simulink model "MultipleAgentsChoice_NoVR"  (Simulink 7.5)
settings: Solver=ode45  StartTime=0.0  StopTime=1000  RelTol=1e-4  AbsTol=1e-4
libraries: simulink x64
(part 5 of 6)

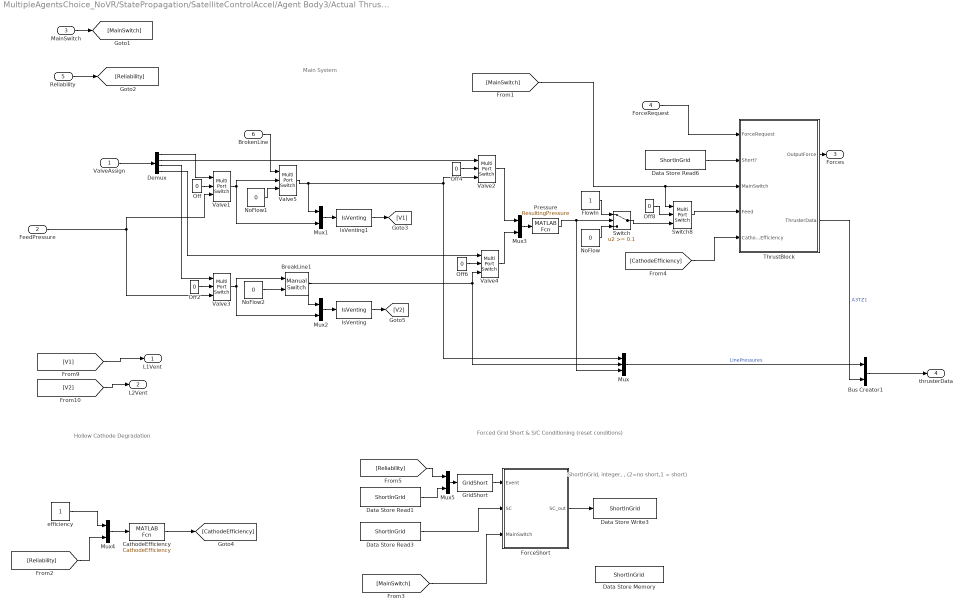
== system MultipleAgentsChoice_NoVR/StatePropagation/SatelliteControlAccel/Agent Body3/Actual Thruster response/Zthruster1/Thruster1 ==
  note: Forced Grid Short & S/C Conditioning (reset conditions)
  note: ShortInGrid, integer, , (2=no short,1 = short)
  note: Hollow Cathode Degradation
  note: Main System
  ValveAssign : Inport  OutDataType=sfix(16)  OutScaling=2^0
  FeedPressure : Inport  Port=2  OutDataType=sfix(16)  OutScaling=2^0
  MainSwitch : Inport  Port=3  OutDataType=sfix(16)  OutScaling=2^0
  ForceRequest : Inport  Port=4  OutDataType=sfix(16)  OutScaling=2^0
  Reliability : Inport  Port=5  OutDataType=sfix(16)  OutScaling=2^0
  BrokenLine : Inport  Port=6  OutDataType=sfix(16)  OutScaling=2^0
  BreakLine1 : simulink/Signal Routing/Manual Switch  SystemSampleTime=-1  sw=1  action=0  varsize=off
  Bus Creator1 : BusCreator  Inputs=2
  CathodeEfficiency : MATLABFcn  MATLABFcn=CathodeEfficiency  OutputDimensions=1
  Data Store Memory : DataStoreMemory  DataStoreName=ShortInGrid  ReadBeforeWriteMsg=warning  WriteAfterWriteMsg=warning  WriteAfterReadMsg=warning  InitialValue=2  OutDataType=sfix(16)  OutScaling=2^0
  Data Store Read1 : DataStoreRead  DataStoreName=ShortInGrid  SampleTime=0
  Data Store Read3 : DataStoreRead  DataStoreName=ShortInGrid  SampleTime=0
  Data Store Read6 : DataStoreRead  DataStoreName=ShortInGrid  SampleTime=0
  Data Store Write3 : DataStoreWrite  DataStoreName=ShortInGrid  SampleTime=-1
  Demux : Demux
  FlowIn : Constant  OutDataType=sfix(16)  OutScaling=2^0
  ForceShort : Subsystem
  GridShort : MATLABFcn  MATLABFcn=GridShort  OutputDimensions=1
  IsVenting : MATLABFcn  MATLABFcn=IsVenting  OutputDimensions=1
  IsVenting1 : MATLABFcn  MATLABFcn=IsVenting  OutputDimensions=1
  Mux : Mux  Inputs=3
  Mux{1..5} (5 alike) : Mux  Inputs=2
  NoFlow : Constant  Value=0  OutDataType=sfix(16)  OutScaling=2^0
  NoFlow1 : Constant  Value=0  OutDataType=sfix(16)  OutScaling=2^0
  NoFlow2 : Constant  Value=0  OutDataType=sfix(16)  OutScaling=2^0
  Off{,2,4,6,8} (5 alike) : Constant  Value=0  OutDataType=sfix(16)  OutScaling=2^0
  Pressure : MATLABFcn  MATLABFcn=ResultingPressure
  Switch : Switch  Threshold=0.1
  Switch8 : MultiPortSwitch  Inputs=2  zeroidx=off
  ThrustBlock : Subsystem
  Valve{1..5} (5 alike) : MultiPortSwitch  Inputs=2  zeroidx=off
  efficiency : Constant  OutDataType=sfix(16)  OutScaling=2^0
  L1Vent : Outport  OutDataType=sfix(16)  OutScaling=2^0
  L2Vent : Outport  Port=2  OutDataType=sfix(16)  OutScaling=2^0
  Forces : Outport  Port=3  OutDataType=sfix(16)  OutScaling=2^0
  thrusterData : Outport  Port=4  OutDataType=sfix(16)  OutScaling=2^0
  wires:
  ForceShort/1(SC_out) -> Data Store Write3/1
  GridShort/1 -> ForceShort/1(Event)
  Data Store Read3/1 -> ForceShort/2(SC)
  [MainSwitch] -> ForceShort/3(MainSwitch)
  Valve1/1 -> Mux1/2, Valve5/2
  Valve2/1 -> Mux3/1
  Mux3/1 -> Pressure/1
  Valve5/1 -> Mux1/1, Valve2/3, Mux/1
  FlowIn/1 -> Switch/1
  NoFlow/1 -> Switch/3
  Switch8/1 -> ThrustBlock/4(Feed)
  Data Store Read6/1 -> ThrustBlock/2(Short?)
  ValveAssign/1 -> Demux/1
  Demux/1 -> Valve1/1
  Demux/2 -> Valve2/1
  Demux/3 -> Valve3/1
  Demux/4 -> Valve4/1
  ThrustBlock/2(ThrusterData) -> Bus Creator1/2  "A3TZ1"
  ThrustBlock/1(OutputForce) -> Forces/1
  NoFlow1/1 -> Valve5/3
  Off/1 -> Valve1/2
  Off4/1 -> Valve2/2
  Off2/1 -> Valve3/2
  Off6/1 -> Valve4/2
  Off8/1 -> Switch8/2
  Switch/1 -> Switch8/3
  Mux/1 -> Bus Creator1/1  "LinePressures"
  NoFlow2/1 -> BreakLine1/2
  Valve3/1 -> BreakLine1/1, Mux2/2
  BreakLine1/1 -> Mux2/1, Valve4/3, Mux/2
  [CathodeEfficiency] -> ThrustBlock/5(CathodeEfficiency)
  ForceRequest/1 -> ThrustBlock/1(ForceRequest)
  Bus Creator1/1 -> thrusterData/1
  Mux1/1 -> IsVenting1/1
  Mux2/1 -> IsVenting/1
  Pressure/1 -> Switch/2, Mux/3
  IsVenting1/1 -> [V1]
  IsVenting/1 -> [V2]
  FeedPressure/1 -> Valve1/3, Valve3/3
  MainSwitch/1 -> [MainSwitch]
  Valve4/1 -> Mux3/2
  [MainSwitch] -> ThrustBlock/3(MainSwitch), Switch8/1
  Reliability/1 -> [Reliability]
  efficiency/1 -> Mux4/1
  [Reliability] -> Mux4/2
  Mux4/1 -> CathodeEfficiency/1
  CathodeEfficiency/1 -> [CathodeEfficiency]
  Mux5/1 -> GridShort/1
  Data Store Read1/1 -> Mux5/2
  [Reliability] -> Mux5/1
  BrokenLine/1 -> Valve5/1
  [V1] -> L1Vent/1
  [V2] -> L2Vent/1

== system MultipleAgentsChoice_NoVR/StatePropagation/SatelliteControlAccel/Agent Body1/Actual Thruster response/XYZthruster/Thruster1/ForceShort ==
  note: Detect event and introduce short, otherwise pass through current result of short status
  Event : Inport  OutDataType=sfix(16)  OutScaling=2^0
  SC : Inport  Port=2  OutDataType=sfix(16)  OutScaling=2^0
  MainSwitch : Inport  Port=3  OutDataType=sfix(16)  OutScaling=2^0
  Constant : Constant  OutDataType=sfix(16)  OutScaling=2^0
  Data Type Conversion : DataTypeConversion  OutDataType=sfix(16)  OutScaling=2^0
  Detect Increase : simulink/Logic and Bit Operations/Detect Increase  SystemSampleTime=-1  vinit=0
  Multiport Switch : MultiPortSwitch  DataPortOrder=Zero-based contiguous  Inputs=2  zeroidx=on
  S/C Conditioning : Subsystem
  SC_out : Outport  OutDataType=sfix(16)  OutScaling=2^0
  wires:
  Event/1 -> Detect Increase/1
  Detect Increase/1 -> Data Type Conversion/1
  S/C Conditioning/1(Short?) -> SC_out/1
  MainSwitch/1 -> S/C Conditioning/2(MainSwitch)
  Data Type Conversion/1 -> Multiport Switch/1
  SC/1 -> Multiport Switch/2
  Constant/1 -> Multiport Switch/3
  Multiport Switch/1 -> S/C Conditioning/1(SC)

== system MultipleAgentsChoice_NoVR/StatePropagation/SatelliteControlAccel/Agent Body1/Actual Thruster response/XYZthruster/Thruster1/ThrustBlock ==
  ForceRequest : Inport  OutDataType=sfix(16)  OutScaling=2^0
  Short? : Inport  Port=2  OutDataType=sfix(16)  OutScaling=2^0
  MainSwitch : Inport  Port=3  OutDataType=sfix(16)  OutScaling=2^0
  Feed : Inport  Port=4  OutDataType=sfix(16)  OutScaling=2^0
  CathodeEfficiency : Inport  Port=5  OutDataType=sfix(16)  OutScaling=2^0
  ActiveThruster (logical) : Subsystem
  Bus Creator : BusCreator  Inputs=2
  Product : Product  OutDataType=sfix(16)  OutScaling=2^0  RndMeth=Zero
  Product1 : Product  OutDataType=sfix(16)  OutScaling=2^0  RndMeth=Zero
  Voltage/Current : Subsystem
  OutputForce : Outport  OutDataType=sfix(16)  OutScaling=2^0
  ThrusterData : Outport  Port=2  OutDataType=sfix(16)  OutScaling=2^0
  wires:
  MainSwitch/1 -> ActiveThruster (logical)/2(ThrusterOn?), Voltage/Current/2(MainSwitch)
  Short?/1 -> ActiveThruster (logical)/1(Short?), Voltage/Current/1(Short?)
  Feed/1 -> Voltage/Current/3(Feed?), ActiveThruster (logical)/3(Feed?)
  Voltage/Current/1(Voltage) -> Bus Creator/1  "voltage"
  Voltage/Current/2(Current) -> Bus Creator/2  "current"
  Bus Creator/1 -> ThrusterData/1
  ActiveThruster (logical)/1(Active) -> Product/1
  ForceRequest/1 -> [ForceRequest]
  CathodeEfficiency/1 -> [CathodeEfficiency]
  Product1/1 -> OutputForce/1
  [ForceRequest] -> Product/2
  Product/1 -> Product1/1
  [CathodeEfficiency] -> Product1/2

== system MultipleAgentsChoice_NoVR/StatePropagation/SatelliteControlAccel/Agent Body1/Actual Thruster response/Xthruster/Thruster1/ForceShort ==
  note: Detect event and introduce short, otherwise pass through current result of short status
  Event : Inport  OutDataType=sfix(16)  OutScaling=2^0
  SC : Inport  Port=2  OutDataType=sfix(16)  OutScaling=2^0
  MainSwitch : Inport  Port=3  OutDataType=sfix(16)  OutScaling=2^0
  Constant : Constant  OutDataType=sfix(16)  OutScaling=2^0
  Data Type Conversion : DataTypeConversion  OutDataType=sfix(16)  OutScaling=2^0
  Detect Increase : simulink/Logic and Bit Operations/Detect Increase  SystemSampleTime=-1  vinit=0
  Multiport Switch : MultiPortSwitch  DataPortOrder=Zero-based contiguous  Inputs=2  zeroidx=on
  S/C Conditioning : Subsystem
  SC_out : Outport  OutDataType=sfix(16)  OutScaling=2^0
  wires:
  Multiport Switch/1 -> S/C Conditioning/1(SC)
  Constant/1 -> Multiport Switch/3
  SC/1 -> Multiport Switch/2
  Data Type Conversion/1 -> Multiport Switch/1
  MainSwitch/1 -> S/C Conditioning/2(MainSwitch)
  S/C Conditioning/1(Short?) -> SC_out/1
  Detect Increase/1 -> Data Type Conversion/1
  Event/1 -> Detect Increase/1

== system MultipleAgentsChoice_NoVR/StatePropagation/SatelliteControlAccel/Agent Body1/Actual Thruster response/Xthruster/Thruster1/ThrustBlock ==
  ForceRequest : Inport  OutDataType=sfix(16)  OutScaling=2^0
  Short? : Inport  Port=2  OutDataType=sfix(16)  OutScaling=2^0
  MainSwitch : Inport  Port=3  OutDataType=sfix(16)  OutScaling=2^0
  Feed : Inport  Port=4  OutDataType=sfix(16)  OutScaling=2^0
  CathodeEfficiency : Inport  Port=5  OutDataType=sfix(16)  OutScaling=2^0
  ActiveThruster (logical) : Subsystem
  Bus Creator : BusCreator  Inputs=2
  Product : Product  OutDataType=sfix(16)  OutScaling=2^0  RndMeth=Zero
  Product1 : Product  OutDataType=sfix(16)  OutScaling=2^0  RndMeth=Zero
  Voltage/Current : Subsystem
  OutputForce : Outport  OutDataType=sfix(16)  OutScaling=2^0
  ThrusterData : Outport  Port=2  OutDataType=sfix(16)  OutScaling=2^0
  wires:
  [CathodeEfficiency] -> Product1/2
  Product/1 -> Product1/1
  [ForceRequest] -> Product/2
  CathodeEfficiency/1 -> [CathodeEfficiency]
  ForceRequest/1 -> [ForceRequest]
  ActiveThruster (logical)/1(Active) -> Product/1
  Bus Creator/1 -> ThrusterData/1
  Voltage/Current/2(Current) -> Bus Creator/2  "current"
  Voltage/Current/1(Voltage) -> Bus Creator/1  "voltage"
  Feed/1 -> ActiveThruster (logical)/3(Feed?), Voltage/Current/3(Feed?)
  Short?/1 -> Voltage/Current/1(Short?), ActiveThruster (logical)/1(Short?)
  MainSwitch/1 -> Voltage/Current/2(MainSwitch), ActiveThruster (logical)/2(ThrusterOn?)
  Product1/1 -> OutputForce/1

== system MultipleAgentsChoice_NoVR/StatePropagation/SatelliteControlAccel/Agent Body1/Actual Thruster response/Ythruster1/Thruster1/ForceShort ==
  note: Detect event and introduce short, otherwise pass through current result of short status
  Event : Inport  OutDataType=sfix(16)  OutScaling=2^0
  SC : Inport  Port=2  OutDataType=sfix(16)  OutScaling=2^0
  MainSwitch : Inport  Port=3  OutDataType=sfix(16)  OutScaling=2^0
  Constant : Constant  OutDataType=sfix(16)  OutScaling=2^0
  Data Type Conversion : DataTypeConversion  OutDataType=sfix(16)  OutScaling=2^0
  Detect Increase : simulink/Logic and Bit Operations/Detect Increase  SystemSampleTime=-1  vinit=0
  Multiport Switch : MultiPortSwitch  DataPortOrder=Zero-based contiguous  Inputs=2  zeroidx=on
  S/C Conditioning : Subsystem
  SC_out : Outport  OutDataType=sfix(16)  OutScaling=2^0
  wires:
  Event/1 -> Detect Increase/1
  Detect Increase/1 -> Data Type Conversion/1
  S/C Conditioning/1(Short?) -> SC_out/1
  MainSwitch/1 -> S/C Conditioning/2(MainSwitch)
  Data Type Conversion/1 -> Multiport Switch/1
  SC/1 -> Multiport Switch/2
  Constant/1 -> Multiport Switch/3
  Multiport Switch/1 -> S/C Conditioning/1(SC)

== system MultipleAgentsChoice_NoVR/StatePropagation/SatelliteControlAccel/Agent Body1/Actual Thruster response/Ythruster1/Thruster1/ThrustBlock ==
  ForceRequest : Inport  OutDataType=sfix(16)  OutScaling=2^0
  Short? : Inport  Port=2  OutDataType=sfix(16)  OutScaling=2^0
  MainSwitch : Inport  Port=3  OutDataType=sfix(16)  OutScaling=2^0
  Feed : Inport  Port=4  OutDataType=sfix(16)  OutScaling=2^0
  CathodeEfficiency : Inport  Port=5  OutDataType=sfix(16)  OutScaling=2^0
  ActiveThruster (logical) : Subsystem
  Bus Creator : BusCreator  Inputs=2
  Product : Product  OutDataType=sfix(16)  OutScaling=2^0  RndMeth=Zero
  Product1 : Product  OutDataType=sfix(16)  OutScaling=2^0  RndMeth=Zero
  Voltage/Current : Subsystem
  OutputForce : Outport  OutDataType=sfix(16)  OutScaling=2^0
  ThrusterData : Outport  Port=2  OutDataType=sfix(16)  OutScaling=2^0
  wires:
  MainSwitch/1 -> ActiveThruster (logical)/2(ThrusterOn?), Voltage/Current/2(MainSwitch)
  Short?/1 -> ActiveThruster (logical)/1(Short?), Voltage/Current/1(Short?)
  Feed/1 -> Voltage/Current/3(Feed?), ActiveThruster (logical)/3(Feed?)
  Voltage/Current/1(Voltage) -> Bus Creator/1  "voltage"
  Voltage/Current/2(Current) -> Bus Creator/2  "current"
  Bus Creator/1 -> ThrusterData/1
  ActiveThruster (logical)/1(Active) -> Product/1
  ForceRequest/1 -> [ForceRequest]
  CathodeEfficiency/1 -> [CathodeEfficiency]
  Product1/1 -> OutputForce/1
  [ForceRequest] -> Product/2
  Product/1 -> Product1/1
  [CathodeEfficiency] -> Product1/2

== system MultipleAgentsChoice_NoVR/StatePropagation/SatelliteControlAccel/Agent Body1/Actual Thruster response/Zthruster1/Thruster1/ForceShort ==
  note: Detect event and introduce short, otherwise pass through current result of short status
  Event : Inport  OutDataType=sfix(16)  OutScaling=2^0
  SC : Inport  Port=2  OutDataType=sfix(16)  OutScaling=2^0
  MainSwitch : Inport  Port=3  OutDataType=sfix(16)  OutScaling=2^0
  Constant : Constant  OutDataType=sfix(16)  OutScaling=2^0
  Data Type Conversion : DataTypeConversion  OutDataType=sfix(16)  OutScaling=2^0
  Detect Increase : simulink/Logic and Bit Operations/Detect Increase  SystemSampleTime=-1  vinit=0
  Multiport Switch : MultiPortSwitch  DataPortOrder=Zero-based contiguous  Inputs=2  zeroidx=on
  S/C Conditioning : Subsystem
  SC_out : Outport  OutDataType=sfix(16)  OutScaling=2^0
  wires:
  Multiport Switch/1 -> S/C Conditioning/1(SC)
  Constant/1 -> Multiport Switch/3
  SC/1 -> Multiport Switch/2
  Data Type Conversion/1 -> Multiport Switch/1
  MainSwitch/1 -> S/C Conditioning/2(MainSwitch)
  S/C Conditioning/1(Short?) -> SC_out/1
  Detect Increase/1 -> Data Type Conversion/1
  Event/1 -> Detect Increase/1

== system MultipleAgentsChoice_NoVR/StatePropagation/SatelliteControlAccel/Agent Body1/Actual Thruster response/Zthruster1/Thruster1/ThrustBlock ==
  ForceRequest : Inport  OutDataType=sfix(16)  OutScaling=2^0
  Short? : Inport  Port=2  OutDataType=sfix(16)  OutScaling=2^0
  MainSwitch : Inport  Port=3  OutDataType=sfix(16)  OutScaling=2^0
  Feed : Inport  Port=4  OutDataType=sfix(16)  OutScaling=2^0
  CathodeEfficiency : Inport  Port=5  OutDataType=sfix(16)  OutScaling=2^0
  ActiveThruster (logical) : Subsystem
  Bus Creator : BusCreator  Inputs=2
  Product : Product  OutDataType=sfix(16)  OutScaling=2^0  RndMeth=Zero
  Product1 : Product  OutDataType=sfix(16)  OutScaling=2^0  RndMeth=Zero
  Voltage/Current : Subsystem
  OutputForce : Outport  OutDataType=sfix(16)  OutScaling=2^0
  ThrusterData : Outport  Port=2  OutDataType=sfix(16)  OutScaling=2^0
  wires:
  [CathodeEfficiency] -> Product1/2
  Product/1 -> Product1/1
  [ForceRequest] -> Product/2
  Product1/1 -> OutputForce/1
  CathodeEfficiency/1 -> [CathodeEfficiency]
  ForceRequest/1 -> [ForceRequest]
  ActiveThruster (logical)/1(Active) -> Product/1
  Bus Creator/1 -> ThrusterData/1
  Voltage/Current/2(Current) -> Bus Creator/2  "current"
  Voltage/Current/1(Voltage) -> Bus Creator/1  "voltage"
  Feed/1 -> ActiveThruster (logical)/3(Feed?), Voltage/Current/3(Feed?)
  Short?/1 -> Voltage/Current/1(Short?), ActiveThruster (logical)/1(Short?)
  MainSwitch/1 -> Voltage/Current/2(MainSwitch), ActiveThruster (logical)/2(ThrusterOn?)

== system MultipleAgentsChoice_NoVR/StatePropagation/SatelliteControlAccel/Agent Body2/Actual Thruster response/XYZthruster/Thruster1/ForceShort ==
  note: Detect event and introduce short, otherwise pass through current result of short status
  Event : Inport  OutDataType=sfix(16)  OutScaling=2^0
  SC : Inport  Port=2  OutDataType=sfix(16)  OutScaling=2^0
  MainSwitch : Inport  Port=3  OutDataType=sfix(16)  OutScaling=2^0
  Constant : Constant  OutDataType=sfix(16)  OutScaling=2^0
  Data Type Conversion : DataTypeConversion  OutDataType=sfix(16)  OutScaling=2^0
  Detect Increase : simulink/Logic and Bit Operations/Detect Increase  SystemSampleTime=-1  vinit=0
  Multiport Switch : MultiPortSwitch  DataPortOrder=Zero-based contiguous  Inputs=2  zeroidx=on
  S/C Conditioning : Subsystem
  SC_out : Outport  OutDataType=sfix(16)  OutScaling=2^0
  wires:
  Multiport Switch/1 -> S/C Conditioning/1(SC)
  Constant/1 -> Multiport Switch/3
  SC/1 -> Multiport Switch/2
  Data Type Conversion/1 -> Multiport Switch/1
  MainSwitch/1 -> S/C Conditioning/2(MainSwitch)
  S/C Conditioning/1(Short?) -> SC_out/1
  Detect Increase/1 -> Data Type Conversion/1
  Event/1 -> Detect Increase/1

== system MultipleAgentsChoice_NoVR/StatePropagation/SatelliteControlAccel/Agent Body2/Actual Thruster response/XYZthruster/Thruster1/ThrustBlock ==
  ForceRequest : Inport  OutDataType=sfix(16)  OutScaling=2^0
  Short? : Inport  Port=2  OutDataType=sfix(16)  OutScaling=2^0
  MainSwitch : Inport  Port=3  OutDataType=sfix(16)  OutScaling=2^0
  Feed : Inport  Port=4  OutDataType=sfix(16)  OutScaling=2^0
  CathodeEfficiency : Inport  Port=5  OutDataType=sfix(16)  OutScaling=2^0
  ActiveThruster (logical) : Subsystem
  Bus Creator : BusCreator  Inputs=2
  Product : Product  OutDataType=sfix(16)  OutScaling=2^0  RndMeth=Zero
  Product1 : Product  OutDataType=sfix(16)  OutScaling=2^0  RndMeth=Zero
  Voltage/Current : Subsystem
  OutputForce : Outport  OutDataType=sfix(16)  OutScaling=2^0
  ThrusterData : Outport  Port=2  OutDataType=sfix(16)  OutScaling=2^0
  wires:
  [CathodeEfficiency] -> Product1/2
  Product/1 -> Product1/1
  [ForceRequest] -> Product/2
  CathodeEfficiency/1 -> [CathodeEfficiency]
  ForceRequest/1 -> [ForceRequest]
  ActiveThruster (logical)/1(Active) -> Product/1
  Bus Creator/1 -> ThrusterData/1
  Voltage/Current/2(Current) -> Bus Creator/2  "current"
  Voltage/Current/1(Voltage) -> Bus Creator/1  "voltage"
  Feed/1 -> ActiveThruster (logical)/3(Feed?), Voltage/Current/3(Feed?)
  Short?/1 -> Voltage/Current/1(Short?), ActiveThruster (logical)/1(Short?)
  MainSwitch/1 -> Voltage/Current/2(MainSwitch), ActiveThruster (logical)/2(ThrusterOn?)
  Product1/1 -> OutputForce/1

== system MultipleAgentsChoice_NoVR/StatePropagation/SatelliteControlAccel/Agent Body2/Actual Thruster response/Xthruster/Thruster1/ForceShort ==
  note: Detect event and introduce short, otherwise pass through current result of short status
  Event : Inport  OutDataType=sfix(16)  OutScaling=2^0
  SC : Inport  Port=2  OutDataType=sfix(16)  OutScaling=2^0
  MainSwitch : Inport  Port=3  OutDataType=sfix(16)  OutScaling=2^0
  Constant : Constant  OutDataType=sfix(16)  OutScaling=2^0
  Data Type Conversion : DataTypeConversion  OutDataType=sfix(16)  OutScaling=2^0
  Detect Increase : simulink/Logic and Bit Operations/Detect Increase  SystemSampleTime=-1  vinit=0
  Multiport Switch : MultiPortSwitch  DataPortOrder=Zero-based contiguous  Inputs=2  zeroidx=on
  S/C Conditioning : Subsystem
  SC_out : Outport  OutDataType=sfix(16)  OutScaling=2^0
  wires:
  Event/1 -> Detect Increase/1
  Detect Increase/1 -> Data Type Conversion/1
  S/C Conditioning/1(Short?) -> SC_out/1
  MainSwitch/1 -> S/C Conditioning/2(MainSwitch)
  Data Type Conversion/1 -> Multiport Switch/1
  SC/1 -> Multiport Switch/2
  Constant/1 -> Multiport Switch/3
  Multiport Switch/1 -> S/C Conditioning/1(SC)

== system MultipleAgentsChoice_NoVR/StatePropagation/SatelliteControlAccel/Agent Body2/Actual Thruster response/Xthruster/Thruster1/ThrustBlock ==
  ForceRequest : Inport  OutDataType=sfix(16)  OutScaling=2^0
  Short? : Inport  Port=2  OutDataType=sfix(16)  OutScaling=2^0
  MainSwitch : Inport  Port=3  OutDataType=sfix(16)  OutScaling=2^0
  Feed : Inport  Port=4  OutDataType=sfix(16)  OutScaling=2^0
  CathodeEfficiency : Inport  Port=5  OutDataType=sfix(16)  OutScaling=2^0
  ActiveThruster (logical) : Subsystem
  Bus Creator : BusCreator  Inputs=2
  Product : Product  OutDataType=sfix(16)  OutScaling=2^0  RndMeth=Zero
  Product1 : Product  OutDataType=sfix(16)  OutScaling=2^0  RndMeth=Zero
  Voltage/Current : Subsystem
  OutputForce : Outport  OutDataType=sfix(16)  OutScaling=2^0
  ThrusterData : Outport  Port=2  OutDataType=sfix(16)  OutScaling=2^0
  wires:
  MainSwitch/1 -> ActiveThruster (logical)/2(ThrusterOn?), Voltage/Current/2(MainSwitch)
  Short?/1 -> ActiveThruster (logical)/1(Short?), Voltage/Current/1(Short?)
  Feed/1 -> Voltage/Current/3(Feed?), ActiveThruster (logical)/3(Feed?)
  Voltage/Current/1(Voltage) -> Bus Creator/1  "voltage"
  Voltage/Current/2(Current) -> Bus Creator/2  "current"
  Bus Creator/1 -> ThrusterData/1
  ActiveThruster (logical)/1(Active) -> Product/1
  ForceRequest/1 -> [ForceRequest]
  CathodeEfficiency/1 -> [CathodeEfficiency]
  [ForceRequest] -> Product/2
  Product/1 -> Product1/1
  [CathodeEfficiency] -> Product1/2
  Product1/1 -> OutputForce/1

== system MultipleAgentsChoice_NoVR/StatePropagation/SatelliteControlAccel/Agent Body2/Actual Thruster response/Ythruster1/Thruster1/ForceShort ==
  note: Detect event and introduce short, otherwise pass through current result of short status
  Event : Inport  OutDataType=sfix(16)  OutScaling=2^0
  SC : Inport  Port=2  OutDataType=sfix(16)  OutScaling=2^0
  MainSwitch : Inport  Port=3  OutDataType=sfix(16)  OutScaling=2^0
  Constant : Constant  OutDataType=sfix(16)  OutScaling=2^0
  Data Type Conversion : DataTypeConversion  OutDataType=sfix(16)  OutScaling=2^0
  Detect Increase : simulink/Logic and Bit Operations/Detect Increase  SystemSampleTime=-1  vinit=0
  Multiport Switch : MultiPortSwitch  DataPortOrder=Zero-based contiguous  Inputs=2  zeroidx=on
  S/C Conditioning : Subsystem
  SC_out : Outport  OutDataType=sfix(16)  OutScaling=2^0
  wires:
  Multiport Switch/1 -> S/C Conditioning/1(SC)
  Constant/1 -> Multiport Switch/3
  SC/1 -> Multiport Switch/2
  Data Type Conversion/1 -> Multiport Switch/1
  MainSwitch/1 -> S/C Conditioning/2(MainSwitch)
  S/C Conditioning/1(Short?) -> SC_out/1
  Detect Increase/1 -> Data Type Conversion/1
  Event/1 -> Detect Increase/1

== system MultipleAgentsChoice_NoVR/StatePropagation/SatelliteControlAccel/Agent Body2/Actual Thruster response/Ythruster1/Thruster1/ThrustBlock ==
  ForceRequest : Inport  OutDataType=sfix(16)  OutScaling=2^0
  Short? : Inport  Port=2  OutDataType=sfix(16)  OutScaling=2^0
  MainSwitch : Inport  Port=3  OutDataType=sfix(16)  OutScaling=2^0
  Feed : Inport  Port=4  OutDataType=sfix(16)  OutScaling=2^0
  CathodeEfficiency : Inport  Port=5  OutDataType=sfix(16)  OutScaling=2^0
  ActiveThruster (logical) : Subsystem
  Bus Creator : BusCreator  Inputs=2
  Product : Product  OutDataType=sfix(16)  OutScaling=2^0  RndMeth=Zero
  Product1 : Product  OutDataType=sfix(16)  OutScaling=2^0  RndMeth=Zero
  Voltage/Current : Subsystem
  OutputForce : Outport  OutDataType=sfix(16)  OutScaling=2^0
  ThrusterData : Outport  Port=2  OutDataType=sfix(16)  OutScaling=2^0
  wires:
  [CathodeEfficiency] -> Product1/2
  Product/1 -> Product1/1
  [ForceRequest] -> Product/2
  CathodeEfficiency/1 -> [CathodeEfficiency]
  ForceRequest/1 -> [ForceRequest]
  ActiveThruster (logical)/1(Active) -> Product/1
  Bus Creator/1 -> ThrusterData/1
  Voltage/Current/2(Current) -> Bus Creator/2  "current"
  Voltage/Current/1(Voltage) -> Bus Creator/1  "voltage"
  Feed/1 -> ActiveThruster (logical)/3(Feed?), Voltage/Current/3(Feed?)
  Short?/1 -> Voltage/Current/1(Short?), ActiveThruster (logical)/1(Short?)
  MainSwitch/1 -> Voltage/Current/2(MainSwitch), ActiveThruster (logical)/2(ThrusterOn?)
  Product1/1 -> OutputForce/1

== system MultipleAgentsChoice_NoVR/StatePropagation/SatelliteControlAccel/Agent Body2/Actual Thruster response/Zthruster1/Thruster1/ForceShort ==
  note: Detect event and introduce short, otherwise pass through current result of short status
  Event : Inport  OutDataType=sfix(16)  OutScaling=2^0
  SC : Inport  Port=2  OutDataType=sfix(16)  OutScaling=2^0
  MainSwitch : Inport  Port=3  OutDataType=sfix(16)  OutScaling=2^0
  Constant : Constant  OutDataType=sfix(16)  OutScaling=2^0
  Data Type Conversion : DataTypeConversion  OutDataType=sfix(16)  OutScaling=2^0
  Detect Increase : simulink/Logic and Bit Operations/Detect Increase  SystemSampleTime=-1  vinit=0
  Multiport Switch : MultiPortSwitch  DataPortOrder=Zero-based contiguous  Inputs=2  zeroidx=on
  S/C Conditioning : Subsystem
  SC_out : Outport  OutDataType=sfix(16)  OutScaling=2^0
  wires:
  Event/1 -> Detect Increase/1
  Detect Increase/1 -> Data Type Conversion/1
  S/C Conditioning/1(Short?) -> SC_out/1
  MainSwitch/1 -> S/C Conditioning/2(MainSwitch)
  Data Type Conversion/1 -> Multiport Switch/1
  SC/1 -> Multiport Switch/2
  Constant/1 -> Multiport Switch/3
  Multiport Switch/1 -> S/C Conditioning/1(SC)

== system MultipleAgentsChoice_NoVR/StatePropagation/SatelliteControlAccel/Agent Body2/Actual Thruster response/Zthruster1/Thruster1/ThrustBlock ==
  ForceRequest : Inport  OutDataType=sfix(16)  OutScaling=2^0
  Short? : Inport  Port=2  OutDataType=sfix(16)  OutScaling=2^0
  MainSwitch : Inport  Port=3  OutDataType=sfix(16)  OutScaling=2^0
  Feed : Inport  Port=4  OutDataType=sfix(16)  OutScaling=2^0
  CathodeEfficiency : Inport  Port=5  OutDataType=sfix(16)  OutScaling=2^0
  ActiveThruster (logical) : Subsystem
  Bus Creator : BusCreator  Inputs=2
  Product : Product  OutDataType=sfix(16)  OutScaling=2^0  RndMeth=Zero
  Product1 : Product  OutDataType=sfix(16)  OutScaling=2^0  RndMeth=Zero
  Voltage/Current : Subsystem
  OutputForce : Outport  OutDataType=sfix(16)  OutScaling=2^0
  ThrusterData : Outport  Port=2  OutDataType=sfix(16)  OutScaling=2^0
  wires:
  MainSwitch/1 -> ActiveThruster (logical)/2(ThrusterOn?), Voltage/Current/2(MainSwitch)
  Short?/1 -> ActiveThruster (logical)/1(Short?), Voltage/Current/1(Short?)
  Feed/1 -> Voltage/Current/3(Feed?), ActiveThruster (logical)/3(Feed?)
  Voltage/Current/1(Voltage) -> Bus Creator/1  "voltage"
  Voltage/Current/2(Current) -> Bus Creator/2  "current"
  Bus Creator/1 -> ThrusterData/1
  ActiveThruster (logical)/1(Active) -> Product/1
  ForceRequest/1 -> [ForceRequest]
  CathodeEfficiency/1 -> [CathodeEfficiency]
  [ForceRequest] -> Product/2
  Product/1 -> Product1/1
  [CathodeEfficiency] -> Product1/2
  Product1/1 -> OutputForce/1

== system MultipleAgentsChoice_NoVR/StatePropagation/SatelliteControlAccel/Agent Body3/Actual Thruster response/XYZthruster/Thruster1/ForceShort ==
  note: Detect event and introduce short, otherwise pass through current result of short status
  Event : Inport  OutDataType=sfix(16)  OutScaling=2^0
  SC : Inport  Port=2  OutDataType=sfix(16)  OutScaling=2^0
  MainSwitch : Inport  Port=3  OutDataType=sfix(16)  OutScaling=2^0
  Constant : Constant  OutDataType=sfix(16)  OutScaling=2^0
  Data Type Conversion : DataTypeConversion  OutDataType=sfix(16)  OutScaling=2^0
  Detect Increase : simulink/Logic and Bit Operations/Detect Increase  SystemSampleTime=-1  vinit=0
  Multiport Switch : MultiPortSwitch  DataPortOrder=Zero-based contiguous  Inputs=2  zeroidx=on
  S/C Conditioning : Subsystem
  SC_out : Outport  OutDataType=sfix(16)  OutScaling=2^0
  wires:
  Multiport Switch/1 -> S/C Conditioning/1(SC)
  Constant/1 -> Multiport Switch/3
  SC/1 -> Multiport Switch/2
  Data Type Conversion/1 -> Multiport Switch/1
  MainSwitch/1 -> S/C Conditioning/2(MainSwitch)
  S/C Conditioning/1(Short?) -> SC_out/1
  Detect Increase/1 -> Data Type Conversion/1
  Event/1 -> Detect Increase/1

== system MultipleAgentsChoice_NoVR/StatePropagation/SatelliteControlAccel/Agent Body3/Actual Thruster response/XYZthruster/Thruster1/ThrustBlock ==
  ForceRequest : Inport  OutDataType=sfix(16)  OutScaling=2^0
  Short? : Inport  Port=2  OutDataType=sfix(16)  OutScaling=2^0
  MainSwitch : Inport  Port=3  OutDataType=sfix(16)  OutScaling=2^0
  Feed : Inport  Port=4  OutDataType=sfix(16)  OutScaling=2^0
  CathodeEfficiency : Inport  Port=5  OutDataType=sfix(16)  OutScaling=2^0
  ActiveThruster (logical) : Subsystem
  Bus Creator : BusCreator  Inputs=2
  Product : Product  OutDataType=sfix(16)  OutScaling=2^0  RndMeth=Zero
  Product1 : Product  OutDataType=sfix(16)  OutScaling=2^0  RndMeth=Zero
  Voltage/Current : Subsystem
  OutputForce : Outport  OutDataType=sfix(16)  OutScaling=2^0
  ThrusterData : Outport  Port=2  OutDataType=sfix(16)  OutScaling=2^0
  wires:
  [CathodeEfficiency] -> Product1/2
  Product/1 -> Product1/1
  [ForceRequest] -> Product/2
  CathodeEfficiency/1 -> [CathodeEfficiency]
  ForceRequest/1 -> [ForceRequest]
  ActiveThruster (logical)/1(Active) -> Product/1
  Bus Creator/1 -> ThrusterData/1
  Voltage/Current/2(Current) -> Bus Creator/2  "current"
  Voltage/Current/1(Voltage) -> Bus Creator/1  "voltage"
  Feed/1 -> ActiveThruster (logical)/3(Feed?), Voltage/Current/3(Feed?)
  Short?/1 -> Voltage/Current/1(Short?), ActiveThruster (logical)/1(Short?)
  MainSwitch/1 -> Voltage/Current/2(MainSwitch), ActiveThruster (logical)/2(ThrusterOn?)
  Product1/1 -> OutputForce/1

== system MultipleAgentsChoice_NoVR/StatePropagation/SatelliteControlAccel/Agent Body3/Actual Thruster response/Xthruster/Thruster1/ForceShort ==
  note: Detect event and introduce short, otherwise pass through current result of short status
  Event : Inport  OutDataType=sfix(16)  OutScaling=2^0
  SC : Inport  Port=2  OutDataType=sfix(16)  OutScaling=2^0
  MainSwitch : Inport  Port=3  OutDataType=sfix(16)  OutScaling=2^0
  Constant : Constant  OutDataType=sfix(16)  OutScaling=2^0
  Data Type Conversion : DataTypeConversion  OutDataType=sfix(16)  OutScaling=2^0
  Detect Increase : simulink/Logic and Bit Operations/Detect Increase  SystemSampleTime=-1  vinit=0
  Multiport Switch : MultiPortSwitch  DataPortOrder=Zero-based contiguous  Inputs=2  zeroidx=on
  S/C Conditioning : Subsystem
  SC_out : Outport  OutDataType=sfix(16)  OutScaling=2^0
  wires:
  Event/1 -> Detect Increase/1
  Detect Increase/1 -> Data Type Conversion/1
  S/C Conditioning/1(Short?) -> SC_out/1
  MainSwitch/1 -> S/C Conditioning/2(MainSwitch)
  Data Type Conversion/1 -> Multiport Switch/1
  SC/1 -> Multiport Switch/2
  Constant/1 -> Multiport Switch/3
  Multiport Switch/1 -> S/C Conditioning/1(SC)

== system MultipleAgentsChoice_NoVR/StatePropagation/SatelliteControlAccel/Agent Body3/Actual Thruster response/Xthruster/Thruster1/ThrustBlock ==
  ForceRequest : Inport  OutDataType=sfix(16)  OutScaling=2^0
  Short? : Inport  Port=2  OutDataType=sfix(16)  OutScaling=2^0
  MainSwitch : Inport  Port=3  OutDataType=sfix(16)  OutScaling=2^0
  Feed : Inport  Port=4  OutDataType=sfix(16)  OutScaling=2^0
  CathodeEfficiency : Inport  Port=5  OutDataType=sfix(16)  OutScaling=2^0
  ActiveThruster (logical) : Subsystem
  Bus Creator : BusCreator  Inputs=2
  Product : Product  OutDataType=sfix(16)  OutScaling=2^0  RndMeth=Zero
  Product1 : Product  OutDataType=sfix(16)  OutScaling=2^0  RndMeth=Zero
  Voltage/Current : Subsystem
  OutputForce : Outport  OutDataType=sfix(16)  OutScaling=2^0
  ThrusterData : Outport  Port=2  OutDataType=sfix(16)  OutScaling=2^0
  wires:
  MainSwitch/1 -> ActiveThruster (logical)/2(ThrusterOn?), Voltage/Current/2(MainSwitch)
  Short?/1 -> ActiveThruster (logical)/1(Short?), Voltage/Current/1(Short?)
  Feed/1 -> Voltage/Current/3(Feed?), ActiveThruster (logical)/3(Feed?)
  Voltage/Current/1(Voltage) -> Bus Creator/1  "voltage"
  Voltage/Current/2(Current) -> Bus Creator/2  "current"
  Bus Creator/1 -> ThrusterData/1
  ActiveThruster (logical)/1(Active) -> Product/1
  ForceRequest/1 -> [ForceRequest]
  CathodeEfficiency/1 -> [CathodeEfficiency]
  [ForceRequest] -> Product/2
  Product/1 -> Product1/1
  [CathodeEfficiency] -> Product1/2
  Product1/1 -> OutputForce/1

== system MultipleAgentsChoice_NoVR/StatePropagation/SatelliteControlAccel/Agent Body3/Actual Thruster response/Ythruster1/Thruster1/ForceShort ==
  note: Detect event and introduce short, otherwise pass through current result of short status
  Event : Inport  OutDataType=sfix(16)  OutScaling=2^0
  SC : Inport  Port=2  OutDataType=sfix(16)  OutScaling=2^0
  MainSwitch : Inport  Port=3  OutDataType=sfix(16)  OutScaling=2^0
  Constant : Constant  OutDataType=sfix(16)  OutScaling=2^0
  Data Type Conversion : DataTypeConversion  OutDataType=sfix(16)  OutScaling=2^0
  Detect Increase : simulink/Logic and Bit Operations/Detect Increase  SystemSampleTime=-1  vinit=0
  Multiport Switch : MultiPortSwitch  DataPortOrder=Zero-based contiguous  Inputs=2  zeroidx=on
  S/C Conditioning : Subsystem
  SC_out : Outport  OutDataType=sfix(16)  OutScaling=2^0
  wires:
  Multiport Switch/1 -> S/C Conditioning/1(SC)
  Constant/1 -> Multiport Switch/3
  SC/1 -> Multiport Switch/2
  Data Type Conversion/1 -> Multiport Switch/1
  MainSwitch/1 -> S/C Conditioning/2(MainSwitch)
  S/C Conditioning/1(Short?) -> SC_out/1
  Detect Increase/1 -> Data Type Conversion/1
  Event/1 -> Detect Increase/1

== system MultipleAgentsChoice_NoVR/StatePropagation/SatelliteControlAccel/Agent Body3/Actual Thruster response/Ythruster1/Thruster1/ThrustBlock ==
  ForceRequest : Inport  OutDataType=sfix(16)  OutScaling=2^0
  Short? : Inport  Port=2  OutDataType=sfix(16)  OutScaling=2^0
  MainSwitch : Inport  Port=3  OutDataType=sfix(16)  OutScaling=2^0
  Feed : Inport  Port=4  OutDataType=sfix(16)  OutScaling=2^0
  CathodeEfficiency : Inport  Port=5  OutDataType=sfix(16)  OutScaling=2^0
  ActiveThruster (logical) : Subsystem
  Bus Creator : BusCreator  Inputs=2
  Product : Product  OutDataType=sfix(16)  OutScaling=2^0  RndMeth=Zero
  Product1 : Product  OutDataType=sfix(16)  OutScaling=2^0  RndMeth=Zero
  Voltage/Current : Subsystem
  OutputForce : Outport  OutDataType=sfix(16)  OutScaling=2^0
  ThrusterData : Outport  Port=2  OutDataType=sfix(16)  OutScaling=2^0
  wires:
  [CathodeEfficiency] -> Product1/2
  Product/1 -> Product1/1
  [ForceRequest] -> Product/2
  CathodeEfficiency/1 -> [CathodeEfficiency]
  ForceRequest/1 -> [ForceRequest]
  ActiveThruster (logical)/1(Active) -> Product/1
  Bus Creator/1 -> ThrusterData/1
  Voltage/Current/2(Current) -> Bus Creator/2  "current"
  Voltage/Current/1(Voltage) -> Bus Creator/1  "voltage"
  Feed/1 -> ActiveThruster (logical)/3(Feed?), Voltage/Current/3(Feed?)
  Short?/1 -> Voltage/Current/1(Short?), ActiveThruster (logical)/1(Short?)
  MainSwitch/1 -> Voltage/Current/2(MainSwitch), ActiveThruster (logical)/2(ThrusterOn?)
  Product1/1 -> OutputForce/1

== system MultipleAgentsChoice_NoVR/StatePropagation/SatelliteControlAccel/Agent Body3/Actual Thruster response/Zthruster1/Thruster1/ForceShort ==
  note: Detect event and introduce short, otherwise pass through current result of short status
  Event : Inport  OutDataType=sfix(16)  OutScaling=2^0
  SC : Inport  Port=2  OutDataType=sfix(16)  OutScaling=2^0
  MainSwitch : Inport  Port=3  OutDataType=sfix(16)  OutScaling=2^0
  Constant : Constant  OutDataType=sfix(16)  OutScaling=2^0
  Data Type Conversion : DataTypeConversion  OutDataType=sfix(16)  OutScaling=2^0
  Detect Increase : simulink/Logic and Bit Operations/Detect Increase  SystemSampleTime=-1  vinit=0
  Multiport Switch : MultiPortSwitch  DataPortOrder=Zero-based contiguous  Inputs=2  zeroidx=on
  S/C Conditioning : Subsystem
  SC_out : Outport  OutDataType=sfix(16)  OutScaling=2^0
  wires:
  Event/1 -> Detect Increase/1
  Detect Increase/1 -> Data Type Conversion/1
  S/C Conditioning/1(Short?) -> SC_out/1
  MainSwitch/1 -> S/C Conditioning/2(MainSwitch)
  Data Type Conversion/1 -> Multiport Switch/1
  SC/1 -> Multiport Switch/2
  Constant/1 -> Multiport Switch/3
  Multiport Switch/1 -> S/C Conditioning/1(SC)

== system MultipleAgentsChoice_NoVR/StatePropagation/SatelliteControlAccel/Agent Body3/Actual Thruster response/Zthruster1/Thruster1/ThrustBlock ==
  ForceRequest : Inport  OutDataType=sfix(16)  OutScaling=2^0
  Short? : Inport  Port=2  OutDataType=sfix(16)  OutScaling=2^0
  MainSwitch : Inport  Port=3  OutDataType=sfix(16)  OutScaling=2^0
  Feed : Inport  Port=4  OutDataType=sfix(16)  OutScaling=2^0
  CathodeEfficiency : Inport  Port=5  OutDataType=sfix(16)  OutScaling=2^0
  ActiveThruster (logical) : Subsystem
  Bus Creator : BusCreator  Inputs=2
  Product : Product  OutDataType=sfix(16)  OutScaling=2^0  RndMeth=Zero
  Product1 : Product  OutDataType=sfix(16)  OutScaling=2^0  RndMeth=Zero
  Voltage/Current : Subsystem
  OutputForce : Outport  OutDataType=sfix(16)  OutScaling=2^0
  ThrusterData : Outport  Port=2  OutDataType=sfix(16)  OutScaling=2^0
  wires:
  MainSwitch/1 -> ActiveThruster (logical)/2(ThrusterOn?), Voltage/Current/2(MainSwitch)
  Short?/1 -> ActiveThruster (logical)/1(Short?), Voltage/Current/1(Short?)
  Feed/1 -> Voltage/Current/3(Feed?), ActiveThruster (logical)/3(Feed?)
  Voltage/Current/1(Voltage) -> Bus Creator/1  "voltage"
  Voltage/Current/2(Current) -> Bus Creator/2  "current"
  Bus Creator/1 -> ThrusterData/1
  ActiveThruster (logical)/1(Active) -> Product/1
  ForceRequest/1 -> [ForceRequest]
  CathodeEfficiency/1 -> [CathodeEfficiency]
  [ForceRequest] -> Product/2
  Product/1 -> Product1/1
  [CathodeEfficiency] -> Product1/2
  Product1/1 -> OutputForce/1

== system MultipleAgentsChoice_NoVR/StatePropagation/SatelliteControlAccel/Agent Body1/Actual Thruster response/XYZthruster/Thruster1/ForceShort/S/C Conditioning ==
  SC : Inport  OutDataType=sfix(16)  OutScaling=2^0
  MainSwitch : Inport  Port=2  OutDataType=sfix(16)  OutScaling=2^0
  Constant : Constant  Value=2  OutDataType=sfix(16)  OutScaling=2^0
  Data Type Conversion : DataTypeConversion  OutDataType=sfix(16)  OutScaling=2^0
  Detect Decrease : simulink/Logic and Bit Operations/Detect Decrease  SystemSampleTime=-1  vinit=0
  Multiport Switch : MultiPortSwitch  DataPortOrder=Zero-based contiguous  Inputs=2  zeroidx=on
  Short? : Outport  OutDataType=sfix(16)  OutScaling=2^0
  wires:
  MainSwitch/1 -> Detect Decrease/1
  Detect Decrease/1 -> Data Type Conversion/1
  Data Type Conversion/1 -> Multiport Switch/1
  SC/1 -> Multiport Switch/2
  Constant/1 -> Multiport Switch/3
  Multiport Switch/1 -> Short?/1

== system MultipleAgentsChoice_NoVR/StatePropagation/SatelliteControlAccel/Agent Body1/Actual Thruster response/XYZthruster/Thruster1/ThrustBlock/ActiveThruster (logical) ==
  Short? : Inport  OutDataType=sfix(16)  OutScaling=2^0
  ThrusterOn? : Inport  Port=2  OutDataType=sfix(16)  OutScaling=2^0
  Feed? : Inport  Port=3  OutDataType=sfix(16)  OutScaling=2^0
  MATLAB Fcn : MATLABFcn  MATLABFcn=ActiveThruster  OutputDimensions=1
  Mux : Mux  Inputs=3
  Active : Outport  OutDataType=sfix(16)  OutScaling=2^0
  wires:
  Short?/1 -> Mux/1
  ThrusterOn?/1 -> Mux/2
  Feed?/1 -> Mux/3
  Mux/1 -> MATLAB Fcn/1
  MATLAB Fcn/1 -> Active/1

== system MultipleAgentsChoice_NoVR/StatePropagation/SatelliteControlAccel/Agent Body1/Actual Thruster response/XYZthruster/Thruster1/ThrustBlock/Voltage/Current ==
  Short? : Inport  OutDataType=sfix(16)  OutScaling=2^0
  MainSwitch : Inport  Port=2  OutDataType=sfix(16)  OutScaling=2^0
  Feed? : Inport  Port=3  OutDataType=sfix(16)  OutScaling=2^0
  Demux : Demux  Outputs=2
  MATLAB Fcn : MATLABFcn  MATLABFcn=ThrusterData  OutputDimensions=2
  Mux : Mux  Inputs=3
  Voltage : Outport  OutDataType=sfix(16)  OutScaling=2^0
  Current : Outport  Port=2  OutDataType=sfix(16)  OutScaling=2^0
  wires:
  Short?/1 -> Mux/1
  MainSwitch/1 -> Mux/2
  Feed?/1 -> Mux/3
  Mux/1 -> MATLAB Fcn/1
  MATLAB Fcn/1 -> Demux/1
  Demux/1 -> Voltage/1
  Demux/2 -> Current/1

== system MultipleAgentsChoice_NoVR/StatePropagation/SatelliteControlAccel/Agent Body1/Actual Thruster response/Xthruster/Thruster1/ForceShort/S/C Conditioning ==
  SC : Inport  OutDataType=sfix(16)  OutScaling=2^0
  MainSwitch : Inport  Port=2  OutDataType=sfix(16)  OutScaling=2^0
  Constant : Constant  Value=2  OutDataType=sfix(16)  OutScaling=2^0
  Data Type Conversion : DataTypeConversion  OutDataType=sfix(16)  OutScaling=2^0
  Detect Decrease : simulink/Logic and Bit Operations/Detect Decrease  SystemSampleTime=-1  vinit=0
  Multiport Switch : MultiPortSwitch  DataPortOrder=Zero-based contiguous  Inputs=2  zeroidx=on
  Short? : Outport  OutDataType=sfix(16)  OutScaling=2^0
  wires:
  Multiport Switch/1 -> Short?/1
  Constant/1 -> Multiport Switch/3
  SC/1 -> Multiport Switch/2
  Data Type Conversion/1 -> Multiport Switch/1
  Detect Decrease/1 -> Data Type Conversion/1
  MainSwitch/1 -> Detect Decrease/1

== system MultipleAgentsChoice_NoVR/StatePropagation/SatelliteControlAccel/Agent Body1/Actual Thruster response/Xthruster/Thruster1/ThrustBlock/ActiveThruster (logical) ==
  Short? : Inport  OutDataType=sfix(16)  OutScaling=2^0
  ThrusterOn? : Inport  Port=2  OutDataType=sfix(16)  OutScaling=2^0
  Feed? : Inport  Port=3  OutDataType=sfix(16)  OutScaling=2^0
  MATLAB Fcn : MATLABFcn  MATLABFcn=ActiveThruster  OutputDimensions=1
  Mux : Mux  Inputs=3
  Active : Outport  OutDataType=sfix(16)  OutScaling=2^0
  wires:
  MATLAB Fcn/1 -> Active/1
  Mux/1 -> MATLAB Fcn/1
  Feed?/1 -> Mux/3
  ThrusterOn?/1 -> Mux/2
  Short?/1 -> Mux/1

== system MultipleAgentsChoice_NoVR/StatePropagation/SatelliteControlAccel/Agent Body1/Actual Thruster response/Xthruster/Thruster1/ThrustBlock/Voltage/Current ==
  Short? : Inport  OutDataType=sfix(16)  OutScaling=2^0
  MainSwitch : Inport  Port=2  OutDataType=sfix(16)  OutScaling=2^0
  Feed? : Inport  Port=3  OutDataType=sfix(16)  OutScaling=2^0
  Demux : Demux  Outputs=2
  MATLAB Fcn : MATLABFcn  MATLABFcn=ThrusterData  OutputDimensions=2
  Mux : Mux  Inputs=3
  Voltage : Outport  OutDataType=sfix(16)  OutScaling=2^0
  Current : Outport  Port=2  OutDataType=sfix(16)  OutScaling=2^0
  wires:
  Demux/2 -> Current/1
  Demux/1 -> Voltage/1
  MATLAB Fcn/1 -> Demux/1
  Mux/1 -> MATLAB Fcn/1
  Feed?/1 -> Mux/3
  MainSwitch/1 -> Mux/2
  Short?/1 -> Mux/1

== system MultipleAgentsChoice_NoVR/StatePropagation/SatelliteControlAccel/Agent Body1/Actual Thruster response/Ythruster1/Thruster1/ForceShort/S/C Conditioning ==
  SC : Inport  OutDataType=sfix(16)  OutScaling=2^0
  MainSwitch : Inport  Port=2  OutDataType=sfix(16)  OutScaling=2^0
  Constant : Constant  Value=2  OutDataType=sfix(16)  OutScaling=2^0
  Data Type Conversion : DataTypeConversion  OutDataType=sfix(16)  OutScaling=2^0
  Detect Decrease : simulink/Logic and Bit Operations/Detect Decrease  SystemSampleTime=-1  vinit=0
  Multiport Switch : MultiPortSwitch  DataPortOrder=Zero-based contiguous  Inputs=2  zeroidx=on
  Short? : Outport  OutDataType=sfix(16)  OutScaling=2^0
  wires:
  MainSwitch/1 -> Detect Decrease/1
  Detect Decrease/1 -> Data Type Conversion/1
  Data Type Conversion/1 -> Multiport Switch/1
  SC/1 -> Multiport Switch/2
  Constant/1 -> Multiport Switch/3
  Multiport Switch/1 -> Short?/1

== system MultipleAgentsChoice_NoVR/StatePropagation/SatelliteControlAccel/Agent Body1/Actual Thruster response/Ythruster1/Thruster1/ThrustBlock/ActiveThruster (logical) ==
  Short? : Inport  OutDataType=sfix(16)  OutScaling=2^0
  ThrusterOn? : Inport  Port=2  OutDataType=sfix(16)  OutScaling=2^0
  Feed? : Inport  Port=3  OutDataType=sfix(16)  OutScaling=2^0
  MATLAB Fcn : MATLABFcn  MATLABFcn=ActiveThruster  OutputDimensions=1
  Mux : Mux  Inputs=3
  Active : Outport  OutDataType=sfix(16)  OutScaling=2^0
  wires:
  Short?/1 -> Mux/1
  ThrusterOn?/1 -> Mux/2
  Feed?/1 -> Mux/3
  Mux/1 -> MATLAB Fcn/1
  MATLAB Fcn/1 -> Active/1

== system MultipleAgentsChoice_NoVR/StatePropagation/SatelliteControlAccel/Agent Body1/Actual Thruster response/Ythruster1/Thruster1/ThrustBlock/Voltage/Current ==
  Short? : Inport  OutDataType=sfix(16)  OutScaling=2^0
  MainSwitch : Inport  Port=2  OutDataType=sfix(16)  OutScaling=2^0
  Feed? : Inport  Port=3  OutDataType=sfix(16)  OutScaling=2^0
  Demux : Demux  Outputs=2
  MATLAB Fcn : MATLABFcn  MATLABFcn=ThrusterData  OutputDimensions=2
  Mux : Mux  Inputs=3
  Voltage : Outport  OutDataType=sfix(16)  OutScaling=2^0
  Current : Outport  Port=2  OutDataType=sfix(16)  OutScaling=2^0
  wires:
  Short?/1 -> Mux/1
  MainSwitch/1 -> Mux/2
  Feed?/1 -> Mux/3
  Mux/1 -> MATLAB Fcn/1
  MATLAB Fcn/1 -> Demux/1
  Demux/1 -> Voltage/1
  Demux/2 -> Current/1

== system MultipleAgentsChoice_NoVR/StatePropagation/SatelliteControlAccel/Agent Body1/Actual Thruster response/Zthruster1/Thruster1/ForceShort/S/C Conditioning ==
  SC : Inport  OutDataType=sfix(16)  OutScaling=2^0
  MainSwitch : Inport  Port=2  OutDataType=sfix(16)  OutScaling=2^0
  Constant : Constant  Value=2  OutDataType=sfix(16)  OutScaling=2^0
  Data Type Conversion : DataTypeConversion  OutDataType=sfix(16)  OutScaling=2^0
  Detect Decrease : simulink/Logic and Bit Operations/Detect Decrease  SystemSampleTime=-1  vinit=0
  Multiport Switch : MultiPortSwitch  DataPortOrder=Zero-based contiguous  Inputs=2  zeroidx=on
  Short? : Outport  OutDataType=sfix(16)  OutScaling=2^0
  wires:
  Multiport Switch/1 -> Short?/1
  Constant/1 -> Multiport Switch/3
  SC/1 -> Multiport Switch/2
  Data Type Conversion/1 -> Multiport Switch/1
  Detect Decrease/1 -> Data Type Conversion/1
  MainSwitch/1 -> Detect Decrease/1

== system MultipleAgentsChoice_NoVR/StatePropagation/SatelliteControlAccel/Agent Body1/Actual Thruster response/Zthruster1/Thruster1/ThrustBlock/ActiveThruster (logical) ==
  Short? : Inport  OutDataType=sfix(16)  OutScaling=2^0
  ThrusterOn? : Inport  Port=2  OutDataType=sfix(16)  OutScaling=2^0
  Feed? : Inport  Port=3  OutDataType=sfix(16)  OutScaling=2^0
  MATLAB Fcn : MATLABFcn  MATLABFcn=ActiveThruster  OutputDimensions=1
  Mux : Mux  Inputs=3
  Active : Outport  OutDataType=sfix(16)  OutScaling=2^0
  wires:
  MATLAB Fcn/1 -> Active/1
  Mux/1 -> MATLAB Fcn/1
  Feed?/1 -> Mux/3
  ThrusterOn?/1 -> Mux/2
  Short?/1 -> Mux/1

== system MultipleAgentsChoice_NoVR/StatePropagation/SatelliteControlAccel/Agent Body1/Actual Thruster response/Zthruster1/Thruster1/ThrustBlock/Voltage/Current ==
  Short? : Inport  OutDataType=sfix(16)  OutScaling=2^0
  MainSwitch : Inport  Port=2  OutDataType=sfix(16)  OutScaling=2^0
  Feed? : Inport  Port=3  OutDataType=sfix(16)  OutScaling=2^0
  Demux : Demux  Outputs=2
  MATLAB Fcn : MATLABFcn  MATLABFcn=ThrusterData  OutputDimensions=2
  Mux : Mux  Inputs=3
  Voltage : Outport  OutDataType=sfix(16)  OutScaling=2^0
  Current : Outport  Port=2  OutDataType=sfix(16)  OutScaling=2^0
  wires:
  Demux/2 -> Current/1
  Demux/1 -> Voltage/1
  MATLAB Fcn/1 -> Demux/1
  Mux/1 -> MATLAB Fcn/1
  Feed?/1 -> Mux/3
  MainSwitch/1 -> Mux/2
  Short?/1 -> Mux/1

== system MultipleAgentsChoice_NoVR/StatePropagation/SatelliteControlAccel/Agent Body2/Actual Thruster response/XYZthruster/Thruster1/ForceShort/S/C Conditioning ==
  SC : Inport  OutDataType=sfix(16)  OutScaling=2^0
  MainSwitch : Inport  Port=2  OutDataType=sfix(16)  OutScaling=2^0
  Constant : Constant  Value=2  OutDataType=sfix(16)  OutScaling=2^0
  Data Type Conversion : DataTypeConversion  OutDataType=sfix(16)  OutScaling=2^0
  Detect Decrease : simulink/Logic and Bit Operations/Detect Decrease  SystemSampleTime=-1  vinit=0
  Multiport Switch : MultiPortSwitch  DataPortOrder=Zero-based contiguous  Inputs=2  zeroidx=on
  Short? : Outport  OutDataType=sfix(16)  OutScaling=2^0
  wires:
  Multiport Switch/1 -> Short?/1
  Constant/1 -> Multiport Switch/3
  SC/1 -> Multiport Switch/2
  Data Type Conversion/1 -> Multiport Switch/1
  Detect Decrease/1 -> Data Type Conversion/1
  MainSwitch/1 -> Detect Decrease/1

== system MultipleAgentsChoice_NoVR/StatePropagation/SatelliteControlAccel/Agent Body2/Actual Thruster response/XYZthruster/Thruster1/ThrustBlock/ActiveThruster (logical) ==
  Short? : Inport  OutDataType=sfix(16)  OutScaling=2^0
  ThrusterOn? : Inport  Port=2  OutDataType=sfix(16)  OutScaling=2^0
  Feed? : Inport  Port=3  OutDataType=sfix(16)  OutScaling=2^0
  MATLAB Fcn : MATLABFcn  MATLABFcn=ActiveThruster  OutputDimensions=1
  Mux : Mux  Inputs=3
  Active : Outport  OutDataType=sfix(16)  OutScaling=2^0
  wires:
  MATLAB Fcn/1 -> Active/1
  Mux/1 -> MATLAB Fcn/1
  Feed?/1 -> Mux/3
  ThrusterOn?/1 -> Mux/2
  Short?/1 -> Mux/1

== system MultipleAgentsChoice_NoVR/StatePropagation/SatelliteControlAccel/Agent Body2/Actual Thruster response/XYZthruster/Thruster1/ThrustBlock/Voltage/Current ==
  Short? : Inport  OutDataType=sfix(16)  OutScaling=2^0
  MainSwitch : Inport  Port=2  OutDataType=sfix(16)  OutScaling=2^0
  Feed? : Inport  Port=3  OutDataType=sfix(16)  OutScaling=2^0
  Demux : Demux  Outputs=2
  MATLAB Fcn : MATLABFcn  MATLABFcn=ThrusterData  OutputDimensions=2
  Mux : Mux  Inputs=3
  Voltage : Outport  OutDataType=sfix(16)  OutScaling=2^0
  Current : Outport  Port=2  OutDataType=sfix(16)  OutScaling=2^0
  wires:
  Demux/2 -> Current/1
  Demux/1 -> Voltage/1
  MATLAB Fcn/1 -> Demux/1
  Mux/1 -> MATLAB Fcn/1
  Feed?/1 -> Mux/3
  MainSwitch/1 -> Mux/2
  Short?/1 -> Mux/1

== system MultipleAgentsChoice_NoVR/StatePropagation/SatelliteControlAccel/Agent Body2/Actual Thruster response/Xthruster/Thruster1/ForceShort/S/C Conditioning ==
  SC : Inport  OutDataType=sfix(16)  OutScaling=2^0
  MainSwitch : Inport  Port=2  OutDataType=sfix(16)  OutScaling=2^0
  Constant : Constant  Value=2  OutDataType=sfix(16)  OutScaling=2^0
  Data Type Conversion : DataTypeConversion  OutDataType=sfix(16)  OutScaling=2^0
  Detect Decrease : simulink/Logic and Bit Operations/Detect Decrease  SystemSampleTime=-1  vinit=0
  Multiport Switch : MultiPortSwitch  DataPortOrder=Zero-based contiguous  Inputs=2  zeroidx=on
  Short? : Outport  OutDataType=sfix(16)  OutScaling=2^0
  wires:
  MainSwitch/1 -> Detect Decrease/1
  Detect Decrease/1 -> Data Type Conversion/1
  Data Type Conversion/1 -> Multiport Switch/1
  SC/1 -> Multiport Switch/2
  Constant/1 -> Multiport Switch/3
  Multiport Switch/1 -> Short?/1

== system MultipleAgentsChoice_NoVR/StatePropagation/SatelliteControlAccel/Agent Body2/Actual Thruster response/Xthruster/Thruster1/ThrustBlock/ActiveThruster (logical) ==
  Short? : Inport  OutDataType=sfix(16)  OutScaling=2^0
  ThrusterOn? : Inport  Port=2  OutDataType=sfix(16)  OutScaling=2^0
  Feed? : Inport  Port=3  OutDataType=sfix(16)  OutScaling=2^0
  MATLAB Fcn : MATLABFcn  MATLABFcn=ActiveThruster  OutputDimensions=1
  Mux : Mux  Inputs=3
  Active : Outport  OutDataType=sfix(16)  OutScaling=2^0
  wires:
  Short?/1 -> Mux/1
  ThrusterOn?/1 -> Mux/2
  Feed?/1 -> Mux/3
  Mux/1 -> MATLAB Fcn/1
  MATLAB Fcn/1 -> Active/1
